simulink model "mis"  (R2020a)
settings: Solver=VariableStepAuto  StartTime=0.0  StopTime=10  RelTol=1e-3
settings Model: Creator=Marco  LastModifiedBy=Marco

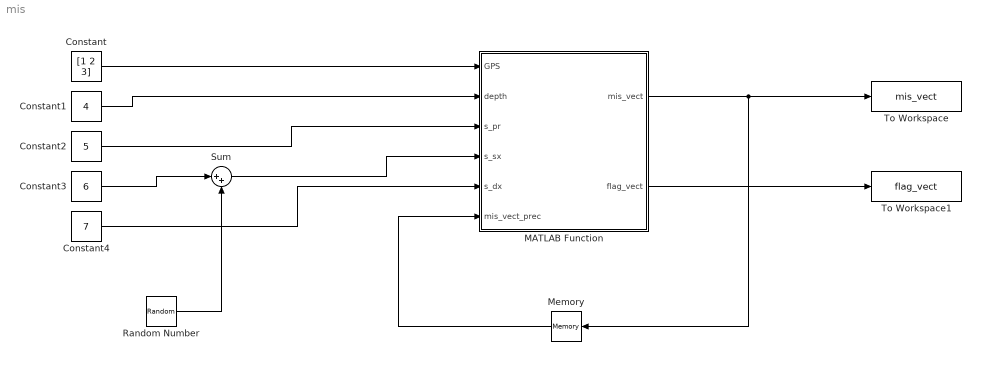
== system mis ==
  Constant : Constant  Value=[1 2 3]
  Constant1 : Constant  Value=4
  Constant2 : Constant  Value=5
  Constant3 : Constant  Value=6
  Constant4 : Constant  Value=7
  MATLAB Function : MATLAB Function  TreatAsAtomicUnit=on
  Memory : Memory
  Random Number : RandomNumber  SampleTime=2
  Sum : Sum  Inputs=|++
  To Workspace : ToWorkspace  VariableName=mis_vect  SaveFormat=Timeseries  SampleTime=-1
  To Workspace1 : ToWorkspace  VariableName=flag_vect  SaveFormat=Timeseries  SampleTime=-1
  wires:
  Constant1/1 -> MATLAB Function/2(depth)
  Constant/1 -> MATLAB Function/1(GPS)
  Constant4/1 -> MATLAB Function/5(s_dx)
  Constant2/1 -> MATLAB Function/3(s_pr)
  MATLAB Function/1(mis_vect) -> To Workspace/1, Memory/1
  Memory/1 -> MATLAB Function/6(mis_vect_prec)
  MATLAB Function/2(flag_vect) -> To Workspace1/1
  Constant3/1 -> Sum/1
  Sum/1 -> MATLAB Function/4(s_sx)
  Random Number/1 -> Sum/2

== matlab function mis/MATLAB Function ==
  data: GPS input; mis_vect output; depth input; s_pr input; s_sx input; s_dx input; mis_vect_prec input; flag_vect output
function [mis_vect,flag_vect] = misure_vector(GPS,depth,s_pr,s_sx,s_dx, mis_vect_prec)
    
    mis_vect = zeros(7,1);
    flag_vect = zeros(7,1);
	mis_vect = [GPS(1) GPS(2) GPS(3) depth s_pr s_sx s_dx]';
    
    for i=[1:7]
        if mis_vect(i) ~= mis_vect_prec(i)
            flag_vect(i) = 1;
        end
    end

end

%{
GPS=[1 2 3];
depth= 4;
s_pr=5;
s_sx=6;
s_dx=7;
%}
